simulink model "heat_exchange_step"  (R2018b)
settings: Solver=ode23s  StartTime=0.0  StopTime=4  RelTol=1e-3
undefined symbols (not defined in the file or in its folder): K, tau, TT
settings Model: Creator=kjartan  LastModifiedBy=kjartan

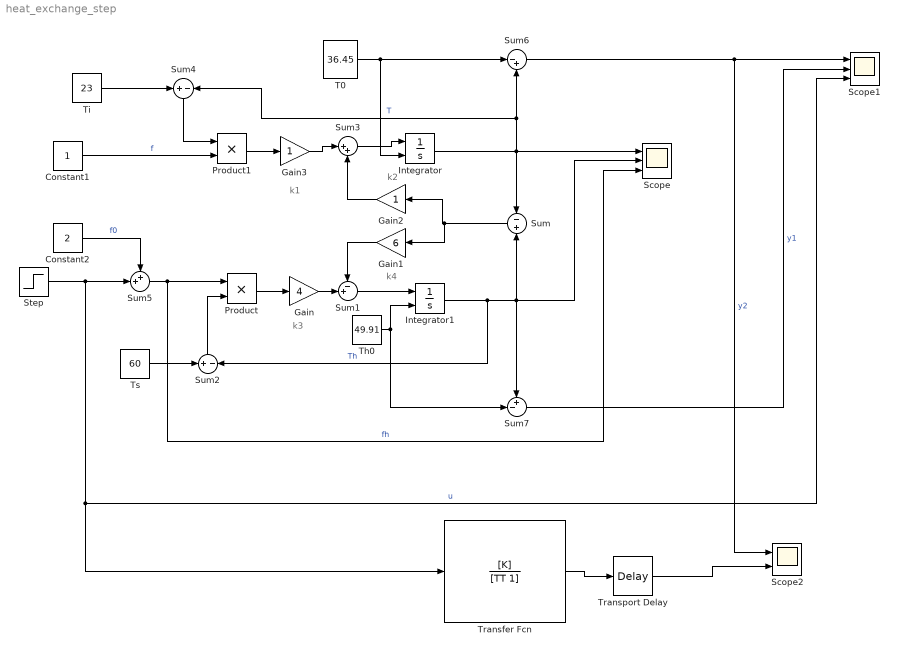
== system heat_exchange_step ==
  note: k3
  note: k4
  note: k2
  note: k1
  Constant1 : Constant
  Constant2 : Constant  Value=2
  Gain : Gain  Gain=4
  Gain1 : Gain  Gain=6
  Gain2 : Gain
  Gain3 : Gain
  Integrator : Integrator  InitialConditionSource=external  InitialCondition=1.4
  Integrator1 : Integrator  InitialConditionSource=external  InitialCondition=1.8
  Product : Product
  Product1 : Product
  Scope : Scope  NumInputPorts=3
  Scope1 : Scope  NumInputPorts=3
  Scope2 : Scope  NumInputPorts=2
  Step : Step  After=2  SampleTime=0
  Sum : Sum  Inputs=-|+
  Sum1 : Sum  Inputs=-+|
  Sum2 : Sum  Inputs=+|-
  Sum3 : Sum  Inputs=|++
  Sum4 : Sum  Inputs=+|-
  Sum5 : Sum  Inputs=++|
  Sum6 : Sum  Inputs=|-+
  Sum7 : Sum  Inputs=+-|
  T0 : Constant  Value=36.45
  Th0 : Constant  Value=49.91
  Ti : Constant  Value=23
  Transfer Fcn : TransferFcn  Numerator=[K]  Denominator=[TT 1]
  Transport Delay : TransportDelay  DelayTime=tau
  Ts : Constant  Value=60
  wires:
  Integrator1/1 -> Sum7/1, Scope/2, Sum/2, Sum2/2  "Th"
  Product/1 -> Gain/1
  Sum1/1 -> Integrator1/1
  Gain/1 -> Sum1/2
  Sum/1 -> Gain1/1, Gain2/1
  Gain1/1 -> Sum1/1
  Ts/1 -> Sum2/1
  Sum2/1 -> Product/2
  Sum3/1 -> Integrator/1
  Gain2/1 -> Sum3/2
  Ti/1 -> Sum4/1
  Sum4/1 -> Product1/1
  Gain3/1 -> Sum3/1
  Step/1 -> Transfer Fcn/1, Scope1/3, Sum5/2  "u"
  Constant2/1 -> Sum5/1  "f0"
  Sum5/1 -> Scope/3, Product/1  "fh"
  T0/1 -> Integrator/2, Sum6/1
  Th0/1 -> Integrator1/2, Sum7/2
  Integrator/1 -> Sum/1, Scope/1, Sum4/2, Sum6/2  "T"
  Sum6/1 -> Scope2/1, Scope1/1  "y2"
  Product1/1 -> Gain3/1
  Constant1/1 -> Product1/2  "f"
  Sum7/1 -> Scope1/2  "y1"
  Transfer Fcn/1 -> Transport Delay/1
  Transport Delay/1 -> Scope2/2
